simulink model "buck_boost__mdl"  (R2018a)
settings: Solver=ode23t  StartTime=0.0  StopTime=5  MaxStep=T_maxStep  RelTol=T_RelTol  AbsTol=T_AbsTol
undefined symbols (not defined in the file): C_out, duty, Ki, Kp, L, R_L, T_sw, Vin
libraries: powerlib x23, simulink x2
settings Model: Creator=Samba_Loks  LastModifiedBy=Samba_Loks

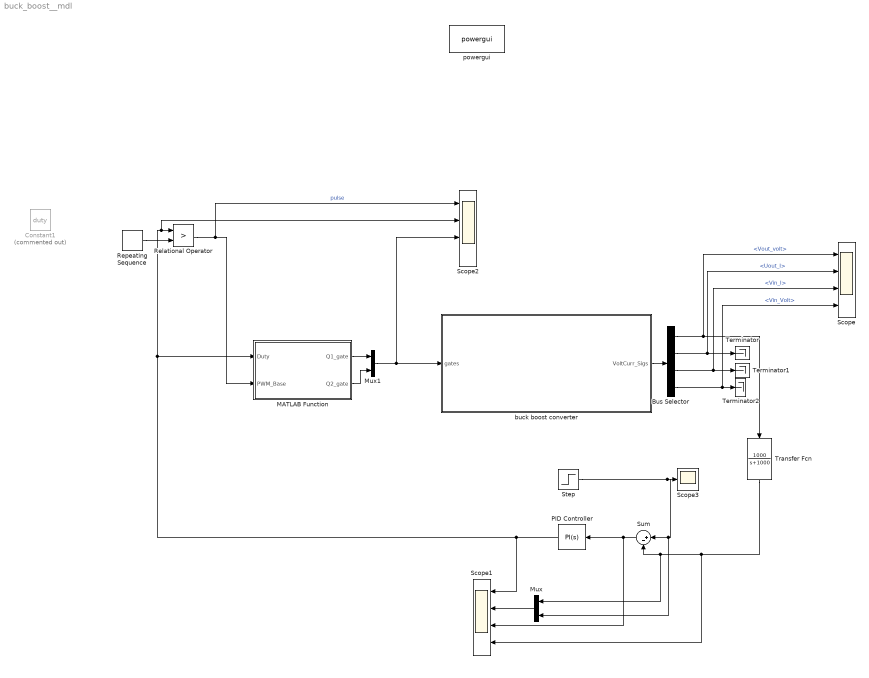
== system buck_boost__mdl ==
  Bus Selector : BusSelector  OutputSignals=Vout_volt,Uout_I,Vin_I,Vin_Volt
  Constant1 : Constant  Commented=on  Value=duty
  MATLAB Function : MATLAB Function  TreatAsAtomicUnit=on
  Mux : Mux  Inputs=2
  Mux1 : Mux  Inputs=2
  PID Controller : simulink/Continuous/PID Controller  Controller=PI  TimeDomain=Continuous-time  SampleTime=-1  IntegratorMethod=Forward Euler  FilterMethod=Forward Euler  Form=Parallel  UseFilter=on  ControllerParametersSource=internal  P=Kp  I=Ki  D=0  N=100  InitialConditionSource=internal  InitialConditionForIntegrator=0  InitialConditionForFilter=0  ExternalReset=none  LimitOutput=off  UpperSaturationLimit=inf  LowerSaturationLimit=-inf  LinearizeAsGain=on  AntiWindupMode=none  Kb=1  TrackingMode=off  Kt=1  PParamMin=[]  PParamMax=[]  IParamMin=[]  IParamMax=[]  DParamMin=[]  DParamMax=[]  NParamMin=[]  NParamMax=[]  KbParamMin=[]  KbParamMax=[]  KtParamMin=[]  KtParamMax=[]  POutMin=[]  POutMax=[]  IOutMin=[]  IOutMax=[]  DOutMin=[]  DOutMax=[]  NOutMin=[]  NOutMax=[]  KbOutMin=[]  KbOutMax=[]  KtOutMin=[]  KtOutMax=[]  IntegratorOutMin=[]  IntegratorOutMax=[]  FilterOutMin=[]  FilterOutMax=[]  SumOutMin=[]  SumOutMax=[]  SumI1OutMin=[]  SumI1OutMax=[]  SumI2OutMin=[]  SumI2OutMax=[]  SumI3OutMin=[]  SumI3OutMax=[]  SumDOutMin=[]  SumDOutMax=[]  SaturationOutMin=[]  SaturationOutMax=[]  IntegratorContinuousStateAttributes=''  IntegratorStateMustResolveToSignalObject=off  IntegratorRTWStateStorageClass=Auto  FilterContinuousStateAttributes=''  FilterStateMustResolveToSignalObject=off  FilterRTWStateStorageClass=Auto  DifferentiatorICPrevScaledInput=0  DifferentiatorOutMin=[]  DifferentiatorOutMax=[]  FilterDiffOutCoefMin=[]  FilterDiffOutCoefMax=[]  SumDenOutMin=[]  SumDenOutMax=[]  SumNumOutMin=[]  SumNumOutMax=[]  ReciprocalOutMin=[]  ReciprocalOutMax=[]  DivideOutMin=[]  DivideOutMax=[]  TunerSelectOption=Transfer Function Based (PID Tuner App)
  Relational Operator : RelationalOperator  Operator=>  OutDataTypeStr=boolean  RndMeth=Simplest
  Repeating Sequence : simulink/Sources/Repeating Sequence  rep_seq_t=[0 T_sw]  rep_seq_y=[0 1]
  Scope : Scope  NumInputPorts=4
  Scope1 : Scope  NumInputPorts=4
  Scope2 : Scope  NumInputPorts=4
  Scope3 : Scope
  Step : Step  Time=0.01  Before=10  After=20  SampleTime=0
  Sum : Sum  Inputs=|+-
  Terminator : Terminator
  Terminator1 : Terminator
  Terminator2 : Terminator
  Transfer Fcn : TransferFcn  Numerator=[1000]  Denominator=[1 1000]
  buck boost converter : Subsystem
  powergui : powerlib/powergui  Priority=1  SimulationMode=Continuous  SampleTime=50e-6  frequency=60  Iterations=50  frequencyindice=0  Pbase=100e6  ErrMax=1e-4  UnitsV=kV  UnitsW=MW  buscounter=0  FunctionMessages=off  echomessages=off  EnableUseOfTLC=off  CurrentSourceSwitches=off  DisableSnubberDevices=off  DisableRonSwitches=off  DisableVfSwitches=off  DisplayEquations=off  SolverType=Tustin/Backward Euler (TBE)  Interpol=off  ExternalGateDelay=off  methode=off  Ts=100  x0status=blocks  SPID=on  SwTol=0  HookPort=off  RestoreLinks=warning  ResistiveCurrentMeasurement=off  Frange=[0:2:500]  Ylog=off  Xlog=on  ShowGrid=off  save=off  variable=ZData  structure=0  ZoomFFT=off  StartTime=0.0  cycles=1  DisplayStyle=1  fundamental=60  FreqAxis=off  MaxFrequency=1000  frequencyindicesteady=1  RmsSteady=1  display=off
  wires:
  Repeating Sequence/1 -> Relational Operator/2
  Relational Operator/1 -> Scope2/1, MATLAB Function/2(PWM_Base)  "pulse"
  MATLAB Function/1(Q1_gate) -> Mux1/1
  MATLAB Function/2(Q2_gate) -> Mux1/2
  Mux1/1 -> Scope2/3, buck boost converter/1(gates)
  buck boost converter/1(VoltCurr_Sigs) -> Bus Selector/1
  Sum/1 -> Scope1/3, PID Controller/1
  Bus Selector/1 -> Transfer Fcn/1, Scope/1  "<Vout_volt>"
  Bus Selector/2 -> Scope/2, Terminator/1  "<Uout_I>"
  Bus Selector/3 -> Scope/3, Terminator1/1  "<Vin_I>"
  Bus Selector/4 -> Scope/4, Terminator2/1  "<Vin_Volt>"
  Step/1 -> Mux/2, Sum/1, Scope3/1
  Mux/1 -> Scope1/2
  PID Controller/1 -> Scope1/1, Scope2/2, Relational Operator/1, MATLAB Function/1(Duty)
  Transfer Fcn/1 -> Scope1/4, Mux/1, Sum/2

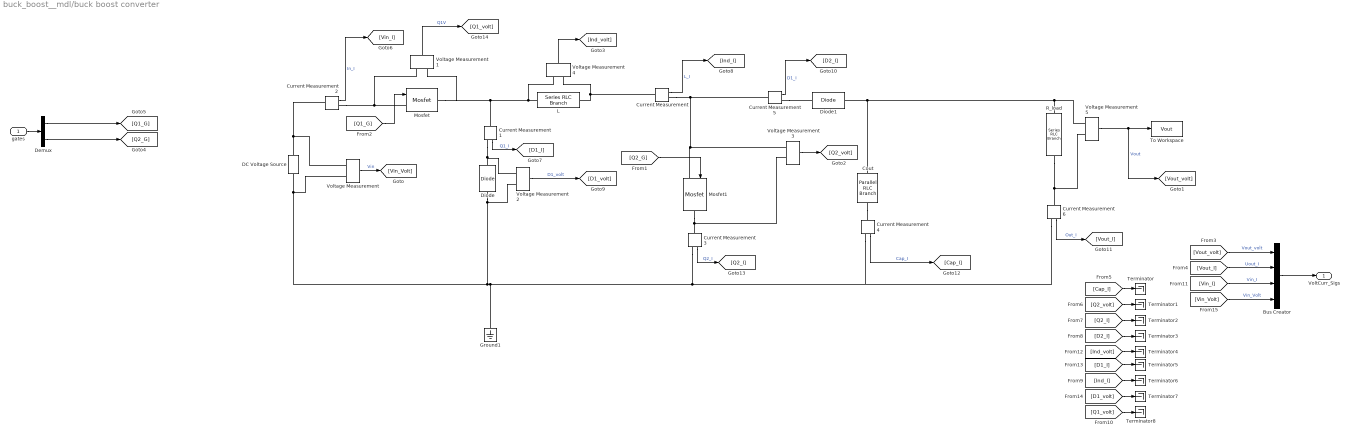
== system buck_boost__mdl/buck boost converter ==
  gates : Inport
  Bus Creator : BusCreator  Inputs=4
  Cout : powerlib/Elements/Parallel RLC Branch  LConnTagsString=a  RConnTagsString=__new0  BranchType=RC  Resistance=inf  Inductance=1e-3  SetiL0=off  InitialCurrent=0  Capacitance=C_out  Setx0=off  InitialVoltage=0  Measurements=None
  Current Measurement{,1..6} (7 alike) : powerlib/Measurements/Current Measurement  PhasorSimulation=off  OutputType=Complex  PSBequivalent=0
  DC Voltage Source : powerlib/Electrical Sources/DC Voltage Source  Amplitude=Vin  Measurements=None
  Demux : Demux  Outputs=2
  Diode : powerlib/Power Electronics/Diode  Ron=0.01  Lon=0  Vf=0.4  IC=0  UseSnubber=0  Rs=500  Cs=250e-9  Measurements=off
  Diode1 : powerlib/Power Electronics/Diode  Ron=0.01  Lon=0  Vf=0.4  IC=0  UseSnubber=0  Rs=500  Cs=250e-9  Measurements=off
  Ground1 : powerlib/Elements/Ground  LConnTagsString=a
  L : powerlib/Elements/Series RLC Branch  LConnTagsString=__new0  RConnTagsString=__new0  BranchType=RL  Resistance=R_L  Inductance=L  SetiL0=off  InitialCurrent=0  Capacitance=1e-6  Setx0=off  InitialVoltage=0  Measurements=None
  Mosfet : powerlib/Power Electronics/Mosfet  Ron=Ron  Lon=0  Rd=R_ds_on  Vfd=V_f_diode  IC=0  Rs=1e5  Cs=inf  Measurements=off
  Mosfet1 : powerlib/Power Electronics/Mosfet  Ron=Ron  Lon=0  Rd=R_ds_on  Vfd=V_f_diode  IC=0  Rs=1e5  Cs=inf  Measurements=off
  R_load : powerlib/Elements/Series RLC Branch  LConnTagsString=__new0  RConnTagsString=__new0  BranchType=RLC  Resistance=5  Inductance=0  SetiL0=off  InitialCurrent=0  Capacitance=inf  Setx0=off  InitialVoltage=0  Measurements=None
  Terminator{,1..8} (9 alike) : Terminator
  To Workspace : ToWorkspace  VariableName=Vout  SampleTime=-1
      settings: Save2DSignal=2-D array (concatenate along first dimension)
  Voltage Measurement{,1..5} (6 alike) : powerlib/Measurements/Voltage Measurement  PhasorSimulation=off  OutputType=Complex  PSBequivalent=0
  VoltCurr_Sigs : Outport
  wires:
  Voltage Measurement5/1 -> [Vout_volt], To Workspace/1  "Vout"
  Voltage Measurement4/1 -> [Ind_volt]
  Current Measurement4/1 -> [Cap_I]  "Cap_I"
  [Q1_G] -> Mosfet/1
  Voltage Measurement/1 -> [Vin_Volt]  "Vin"
  Current Measurement2/1 -> [Vin_I]  "In_I"
  Voltage Measurement3/1 -> [Q2_volt]
  Voltage Measurement2/1 -> [D1_volt]  "D1_volt"
  Current Measurement/1 -> [Ind_I]  "L_I"
  Current Measurement5/1 -> [D2_I]  "D1_I"
  [Q2_G] -> Mosfet1/1
  Voltage Measurement1/1 -> [Q1_volt]  "Q1V"
  Current Measurement1/1 -> [D1_I]  "Q1_I"
  Current Measurement3/1 -> [Q2_I]  "Q2_I"
  Current Measurement6/1 -> [Vout_I]  "Out_I"
  [Cap_I] -> Terminator/1
  [Q2_volt] -> Terminator1/1
  [Q2_I] -> Terminator2/1
  [D2_I] -> Terminator3/1
  [Ind_volt] -> Terminator4/1
  [D1_I] -> Terminator5/1
  [Ind_I] -> Terminator6/1
  [D1_volt] -> Terminator7/1
  [Q1_volt] -> Terminator8/1
  [Vout_volt] -> Bus Creator/1  "Vout_volt"
  [Vout_I] -> Bus Creator/2  "Uout_I"
  [Vin_I] -> Bus Creator/3  "Vin_I"
  [Vin_Volt] -> Bus Creator/4  "Vin_Volt"
  Bus Creator/1 -> VoltCurr_Sigs/1
  Demux/1 -> [Q1_G]
  Demux/2 -> [Q2_G]
  gates/1 -> Demux/1
  connections:
  Voltage Measurement4/LConn1 -- Current Measurement1/LConn1 -- Voltage Measurement1/LConn2 -- Mosfet/RConn1 -- L/LConn1
  R_load/RConn1 -- Voltage Measurement5/LConn2 -- Current Measurement6/LConn1
  Diode/RConn1 -- Voltage Measurement2/LConn1 -- Current Measurement1/RConn1
  Voltage Measurement4/LConn2 -- L/RConn1 -- Current Measurement/LConn1
  Diode/LConn1 -- Voltage Measurement2/LConn2 -- Current Measurement6/RConn1 -- Current Measurement4/RConn1 -- Current Measurement3/RConn1 -- Ground1/LConn1 -- Voltage Measurement/LConn2 -- DC Voltage Source/LConn1
  Voltage Measurement3/LConn1 -- Mosfet1/LConn1 -- Current Measurement5/LConn1 -- Current Measurement/RConn1
  Current Measurement3/LConn1 -- Mosfet1/RConn1 -- Voltage Measurement3/LConn2
  Mosfet/LConn1 -- Current Measurement2/RConn1 -- Voltage Measurement1/LConn1
  Voltage Measurement/LConn1 -- Current Measurement2/LConn1 -- DC Voltage Source/RConn1
  R_load/LConn1 -- Voltage Measurement5/LConn1 -- Diode1/RConn1 -- Cout/LConn1
  Cout/RConn1 -- Current Measurement4/LConn1
  Current Measurement5/RConn1 -- Diode1/LConn1

== matlab function buck_boost__mdl/MATLAB Function ==
  data: Duty input; Q1_gate output; PWM_Base input; Q2_gate output
function [Q1_gate, Q2_gate] = buck_boost_mode_selector(Duty, PWM_Base)
    % Outputs are boolean (true/false)
    
    BUCK_THRESHOLD = 0.48;
    BOOST_THRESHOLD = 0.52;
    
    if Duty < BUCK_THRESHOLD
        % BUCK MODE
        Q1_gate = (PWM_Base ~= 0);  % Convert to boolean
        Q2_gate = false;              % Boolean true
    elseif Duty > BOOST_THRESHOLD
        % BOOST MODE
        Q1_gate = true;
        Q2_gate = (PWM_Base ~= 0);
    else
        % PASS-THROUGH
        Q1_gate = true;
        Q2_gate = false;
    end
end
